simulink model "Mech_sys_nl_obs_deformation"  (R2025b)
settings: Solver=ode15s  StartTime=0.0  StopTime=10.0  RelTol=1e-3
values from neighbouring files (symbols this model uses):
  p_0 = 0    [Init_Simulink_param.m]
  phat_0 = 1e-3    (= 0.001)    [Init_Simulink_param.m]
  q_0 = 0    [Init_Simulink_param.m]
  qhat_0 = 2e-4    (= 0.0002)    [Init_Simulink_param.m]
undefined symbols (not defined in the file or in its folder): params
settings Model: Creator=filippougolini  LastModifiedBy=filippougolini

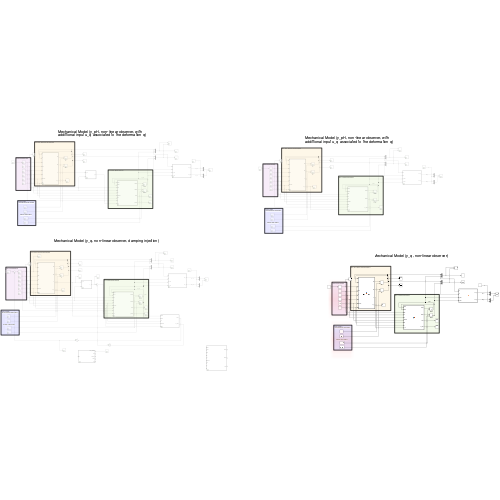
[thumbnail: Simulink's stored preview of the top-level diagram]
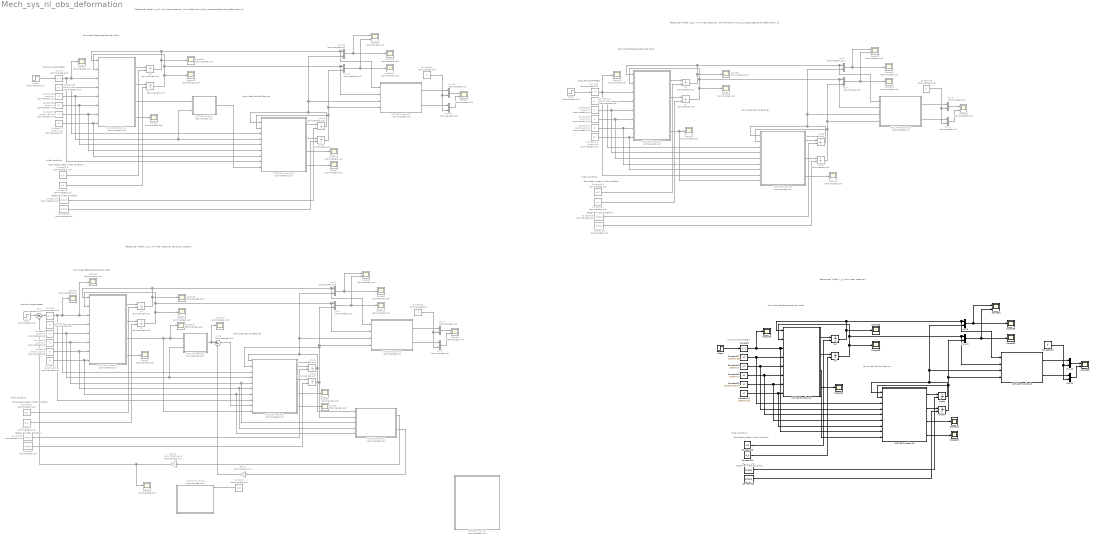
== system Mech_sys_nl_obs_deformation ==
  note: Non-linear Electromechanical plant
  note: Observer initial condition
  note: Non-Linear Spirito Oberver
  note: NonLinear system initial condition
  note: Mechanical Model (y_pH, non-linear observer, with addittional input u_q associated to the deformation q)
  note: Input and parameters
  note: Initial condition
  note: Mechanical Model (y_q, non-linear observer, damping injection)
  note: Non-Linear Spirito Oberver
  note: NonLinear system initial condition
  note: Input and parameters
  note: Initial condition
  note: Non-linear Electromechanical plant
  note: Observer initial condition
  note: Mechanical Model (y_pH, non-linear observer, with addittional input u_q associated to the deformation q)
  note: Non-Linear Spirito Oberver
  note: NonLinear system initial condition
  note: Input and parameters
  note: Initial condition
  note: Non-linear Electromechanical plant
  note: Observer initial condition
  note: NonLinear system initial condition
  note: Non-Linear Spirito Oberver
  note: Observer initial condition
  note: Non-linear Electromechanical plant
  note: Initial condition
  note: Mechanical Model (y_q, non-linear observer)
  note: Input and parameters
  Constant : Constant  Commented=on  Value=100
  Constant1 : Constant  Commented=on  Value=params.q0
  Constant10 : Constant  Commented=on  Value=params.m
  Constant11 : Constant  Commented=on  Value=params.q0
  Constant12 : Constant  Commented=on  Value=params.epsllon
  Constant13 : Constant  Commented=on  Value=q_0
  Constant14 : Constant  Commented=on  Value=p_0
  Constant15 : Constant  Commented=on  Value=qhat_0
  Constant16 : Constant  Commented=on  Value=phat_0
  Constant17 : Constant  Commented=on  Value=params.eta
  Constant18 : Constant  Commented=on  Value=0
  Constant19 : Constant  Commented=on  Value=params.K
  Constant2 : Constant  Commented=on  Value=params.epsllon
  Constant20 : Constant  Commented=on  Value=params.m
  Constant21 : Constant  Value=params.q0
  Constant22 : Constant  Value=params.epsllon
  Constant23 : Constant  Value=q_0
  Constant24 : Constant  Value=p_0
  Constant25 : Constant  Value=qhat_0
  Constant26 : Constant  Value=phat_0
  Constant27 : Constant  Value=params.eta
  Constant28 : Constant  Value=0
  Constant29 : Constant  Value=params.K
  Constant3 : Constant  Commented=on  Value=q_0
  Constant30 : Constant  Value=params.m
  Constant4 : Constant  Commented=on  Value=p_0
  Constant5 : Constant  Commented=on  Value=qhat_0
  Constant6 : Constant  Commented=on  Value=phat_0
  Constant7 : Constant  Commented=on  Value=10
  Constant71 : Constant  Commented=on  Value=params.q0
  Constant74 : Constant  Commented=on  Value=params.epsllon
  Constant76 : Constant  Commented=on  Value=q_0
  Constant77 : Constant  Commented=on  Value=p_0
  Constant79 : Constant  Commented=on  Value=qhat_0
  Constant8 : Constant  Commented=on  Value=0
  Constant80 : Constant  Commented=on  Value=phat_0
  Constant85 : Constant  Commented=on  Value=params.eta
  Constant9 : Constant  Commented=on  Value=params.K
  Constant90 : Constant  Commented=on  Value=0
  Constant92 : Constant  Commented=on  Value=params.K
  Constant93 : Constant  Commented=on  Value=params.m
  Gain1 : Gain  Commented=on  Gain=0
  Gain2 : Gain  Commented=on  Gain=4.957213974e13
  MATLAB Function : MATLAB Function  Commented=on  TreatAsAtomicUnit=on
  MATLAB Function1 : MATLAB Function  Commented=on  TreatAsAtomicUnit=on
  MATLAB Function10 : MATLAB Function  Commented=on  TreatAsAtomicUnit=on
  MATLAB Function12 : MATLAB Function  TreatAsAtomicUnit=on
  MATLAB Function13 : MATLAB Function  TreatAsAtomicUnit=on
  MATLAB Function14 : MATLAB Function  Commented=on  TreatAsAtomicUnit=on
  MATLAB Function15 : MATLAB Function  TreatAsAtomicUnit=on
  MATLAB Function18 : MATLAB Function  Commented=on  TreatAsAtomicUnit=on
  MATLAB Function2 : MATLAB Function  Commented=on  TreatAsAtomicUnit=on
  MATLAB Function22 : MATLAB Function  Commented=on  TreatAsAtomicUnit=on
  MATLAB Function3 : MATLAB Function  Commented=on  TreatAsAtomicUnit=on
  MATLAB Function4 : MATLAB Function  Commented=on  TreatAsAtomicUnit=on
  MATLAB Function5 : MATLAB Function  Commented=on  TreatAsAtomicUnit=on
  MATLAB Function6 : MATLAB Function  Commented=on  TreatAsAtomicUnit=on
  MATLAB Function7 : MATLAB Function  Commented=on  TreatAsAtomicUnit=on
  MATLAB Function8 : MATLAB Function  Commented=on  TreatAsAtomicUnit=on
  MATLAB Function9 : MATLAB Function  Commented=on  TreatAsAtomicUnit=on
  Mux{1..8,39..40,44,46} (12 alike) : Mux  Commented=on  Inputs=2
  Mux{9..12} (4 alike) : Mux  Inputs=2
  Scope{1..7,9..10,12..19,21..22,24..25,27..28,43..44,52..53} (27 alike) : Scope  Commented=on
      Scope1 settings: ActiveDisplayYMinimum=-1  ActiveDisplayYMaximum=1
      Scope10 settings: ActiveDisplayYMinimum=-1  ActiveDisplayYMaximum=1  DataLoggingVariableName=ScopeData3
      Scope12 settings: ActiveDisplayYMinimum=-4.0944874698701246E-5  ActiveDisplayYMaximum=0.0003685038722883113  DataLoggingVariableName=ScopeData5
      Scope13 settings: ActiveDisplayYMinimum=999.83794210721385  ActiveDisplayYMaximum=1000.4797286758781  DataLoggingVariableName=ScopeData12
      Scope14 settings: ActiveDisplayYMinimum=-1  ActiveDisplayYMaximum=1  DataLoggingVariableName=ScopeData6
      Scope15 settings: ActiveDisplayYMinimum=2.4999952064993516E+7  ActiveDisplayYMaximum=2.5000040184962828E+7  DataLoggingVariableName=ScopeData14
      Scope16 settings: ActiveDisplayYMinimum=-3.6994045804858762E+6  ActiveDisplayYMaximum=3.9014912238323367E+6  DataLoggingVariableName=ScopeData15
      Scope17 settings: ActiveDisplayYMinimum=-4.9067926815122174E-14  ActiveDisplayYMaximum=5.0932073184877836E-14  DataLoggingVariableName=ScopeData16
      Scope18 settings: ActiveDisplayYMinimum=-1  ActiveDisplayYMaximum=1  DataLoggingVariableName=ScopeData17
      Scope19 settings: ActiveDisplayYMinimum=-1  ActiveDisplayYMaximum=1  DataLoggingVariableName=ScopeData18
      Scope2 settings: ActiveDisplayYMinimum=-4.486759019288802E-5  ActiveDisplayYMaximum=0.00036893672106914937
      Scope21 settings: ActiveDisplayYMinimum=-4.486759019288802E-5  ActiveDisplayYMaximum=0.00036893672106914937  DataLoggingVariableName=ScopeData20
      Scope22 settings: ActiveDisplayYMinimum=0.000327102944393571  ActiveDisplayYMaximum=0.00032809892974007158  DataLoggingVariableName=ScopeData21
      Scope24 settings: ActiveDisplayYMinimum=-4.4929456410290065E-5  ActiveDisplayYMaximum=0.00036894675529116814  DataLoggingVariableName=ScopeData23
      Scope25 settings: ActiveDisplayYMinimum=-1  ActiveDisplayYMaximum=1  DataLoggingVariableName=ScopeData24
      Scope27 settings: ActiveDisplayYMinimum=-4.0944874698701246E-5  ActiveDisplayYMaximum=0.0003685038722883113  DataLoggingVariableName=ScopeData26
      Scope28 settings: ActiveDisplayYMinimum=-1  ActiveDisplayYMaximum=1  DataLoggingVariableName=ScopeData27
      Scope3 settings: ActiveDisplayYMinimum=-1  ActiveDisplayYMaximum=1  DataLoggingVariableName=ScopeData2
      Scope4 settings: ActiveDisplayYMinimum=-1  ActiveDisplayYMaximum=1  DataLoggingVariableName=ScopeData7
      Scope43 settings: ActiveDisplayYMinimum=-4.4929456410290065E-5  ActiveDisplayYMaximum=0.00036894675529116814  DataLoggingVariableName=ScopeData43
      Scope44 settings: ActiveDisplayYMinimum=-1  ActiveDisplayYMaximum=1  DataLoggingVariableName=ScopeData44
      Scope5 settings: ActiveDisplayYMinimum=-3.6994045804858764E-11  ActiveDisplayYMaximum=3.9014912238323363E-11  DataLoggingVariableName=ScopeData8
      Scope52 settings: ActiveDisplayYMinimum=-4.0944874698701246E-5  ActiveDisplayYMaximum=0.0003685038722883113  DataLoggingVariableName=ScopeData52
      Scope53 settings: ActiveDisplayYMinimum=-1  ActiveDisplayYMaximum=1  DataLoggingVariableName=ScopeData53
      Scope6 settings: ActiveDisplayYMinimum=-4.486759019288802E-5  ActiveDisplayYMaximum=0.00036893672106914937  DataLoggingVariableName=ScopeData9
      Scope7 settings: ActiveDisplayYMinimum=-1  ActiveDisplayYMaximum=1  DataLoggingVariableName=ScopeData10
      Scope9 settings: ActiveDisplayYMinimum=-4.4929456410290065E-5  ActiveDisplayYMaximum=0.00036894675529116814  DataLoggingVariableName=ScopeData13
  Scope{8,11,23,26,37,47} (6 alike) : Scope  Commented=on  NumInputPorts=2
      Scope11 settings: ActiveDisplayYMinimum=-1.6721224120479319E-8  ActiveDisplayYMaximum=1.6255351844579E-8  DataLoggingVariableName=ScopeData4
      Scope23 settings: ActiveDisplayYMinimum=-0.0031018408255779882  ActiveDisplayYMaximum=0.0026704507247831775  DataLoggingVariableName=ScopeData22
      Scope26 settings: ActiveDisplayYMinimum=-0.0014405764588177341  ActiveDisplayYMaximum=0.0029651881293596056  DataLoggingVariableName=ScopeData25
      Scope37 settings: ActiveDisplayYMinimum=-0.0033069856482364551  ActiveDisplayYMaximum=0.0026922054561645506  DataLoggingVariableName=ScopeData37
      Scope47 settings: ActiveDisplayYMinimum=-0.0014633833172245443  ActiveDisplayYMaximum=0.0031704498550208992  DataLoggingVariableName=ScopeData47
      Scope8 settings: ActiveDisplayYMinimum=-0.0048034948171394934  ActiveDisplayYMaximum=0.0043294231290401794  DataLoggingVariableName=ScopeData11
  Scope{20,29..31,33..34,36,38} (8 alike) : Scope
      Scope20 settings: ActiveDisplayYMinimum=-1  ActiveDisplayYMaximum=1  DataLoggingVariableName=ScopeData19
      Scope29 settings: ActiveDisplayYMinimum=-2.6358030258124043E-11  ActiveDisplayYMaximum=1.925982917121927E-11  DataLoggingVariableName=ScopeData28
      Scope30 settings: ActiveDisplayYMinimum=0.0003271907516113819  ActiveDisplayYMaximum=0.00032820530698062  DataLoggingVariableName=ScopeData29
      Scope31 settings: ActiveDisplayYMinimum=-4.0944150570938618E-5  ActiveDisplayYMaximum=0.00036849735513844764  DataLoggingVariableName=ScopeData30
      Scope33 settings: ActiveDisplayYMinimum=-4.4929456410290065E-5  ActiveDisplayYMaximum=0.00036894675529116814  DataLoggingVariableName=ScopeData32
      Scope34 settings: ActiveDisplayYMinimum=-1  ActiveDisplayYMaximum=1  DataLoggingVariableName=ScopeData33
      Scope36 settings: ActiveDisplayYMinimum=0.00032749819334930381  ActiveDisplayYMaximum=0.0003276391478829251  DataLoggingVariableName=ScopeData35
      Scope38 settings: ActiveDisplayYMinimum=-1  ActiveDisplayYMaximum=1  DataLoggingVariableName=ScopeData36
  Scope32 : Scope  NumInputPorts=2
      settings: ActiveDisplayYMinimum=-0.0033241234591442474  ActiveDisplayYMaximum=0.0028464455936065003  DataLoggingVariableName=ScopeData31
  Scope35 : Scope  NumInputPorts=2
      settings: ActiveDisplayYMinimum=-0.0014633833192336466  ActiveDisplayYMaximum=0.0031704498731028193  DataLoggingVariableName=ScopeData34
  Square : Math  Commented=on  Operator=square
  Square1 : Math  Commented=on  Operator=square
  Square2 : Math  Commented=on  Operator=square
  Square3 : Math  Operator=square
  Step1 : Step  Commented=on  After=5e3  SampleTime=0
  Step2 : Step  Commented=on  After=5e3  SampleTime=0
  Step3 : Step  Commented=on  After=5e3  SampleTime=0
  Step4 : Step  After=5e3  SampleTime=0
  Sum : Sum  Commented=on  Inputs=|+-
  Sum1 : Sum  Commented=on  Inputs=|+-
  p1 : Integrator  Commented=on  InitialConditionSource=external
  p2 : Integrator  Commented=on  InitialConditionSource=external
  p3 : Integrator  Commented=on  InitialConditionSource=external
  p4 : Integrator  InitialConditionSource=external
  phat1 : Integrator  Commented=on  InitialConditionSource=external  InitialCondition=5e-4
  phat2 : Integrator  Commented=on  InitialConditionSource=external  InitialCondition=5e-4
  phat3 : Integrator  Commented=on  InitialConditionSource=external  InitialCondition=5e-4
  phat4 : Integrator  InitialConditionSource=external  InitialCondition=5e-4
  q1 : Integrator  Commented=on  InitialConditionSource=external
  q2 : Integrator  Commented=on  InitialConditionSource=external
  q3 : Integrator  Commented=on  InitialConditionSource=external
  q4 : Integrator  InitialConditionSource=external
  qhat1 : Integrator  Commented=on  InitialConditionSource=external  InitialCondition=20e-5
  qhat2 : Integrator  Commented=on  InitialConditionSource=external  InitialCondition=20e-5
  qhat3 : Integrator  Commented=on  InitialConditionSource=external  InitialCondition=20e-5
  qhat4 : Integrator  InitialConditionSource=external  InitialCondition=20e-5
  wires:
  Step3/1 -> Square/1
  MATLAB Function18/3(yhat) -> Scope13/1
  MATLAB Function14/3(y) -> MATLAB Function/1(y_ph)
  Constant80/1 -> phat3/2
  Mux39/1 -> Scope37/1, Scope43/1
  Mux46/1 -> Scope47/1
  Mux40/1 -> Scope37/2, Scope44/1
  phat3/1 -> Mux40/2, MATLAB Function22/4(p_hat), MATLAB Function18/2(phat)  "p_hat"
  Constant93/1 -> MATLAB Function18/5(m), MATLAB Function14/6(m)
  MATLAB Function22/1(err_q) -> Mux46/1  "err_q"
  Constant79/1 -> qhat3/2
  Constant71/1 -> MATLAB Function18/7(q0), MATLAB Function14/8(q0)
  Constant92/1 -> MATLAB Function/2(K), MATLAB Function18/4(K), MATLAB Function14/5(K)
  Constant77/1 -> p3/2
  qhat3/1 -> Mux39/2, MATLAB Function22/3(q_hat), MATLAB Function18/1(qhat)  "q_hat"
  MATLAB Function18/2(dphat) -> phat3/1
  Constant85/1 -> MATLAB Function18/3(eta), MATLAB Function14/4(eta)
  Mux44/1 -> Scope47/2
  MATLAB Function14/1(dq) -> q3/1
  p3/1 -> Scope53/1, Mux40/1, MATLAB Function22/2(p), MATLAB Function14/2(p)  "p"
  MATLAB Function22/2(err_p) -> Mux44/1  "err_p"
  q3/1 -> Scope52/1, Mux39/1, MATLAB Function22/1(q), MATLAB Function14/1(q)  "q"
  MATLAB Function18/1(dqhat) -> qhat3/1
  Constant90/1 -> Mux44/2, Mux46/2  "0"
  Constant76/1 -> q3/2
  Constant74/1 -> MATLAB Function18/6(epsllon), MATLAB Function14/7(epsllon)
  MATLAB Function14/2(dp) -> p3/1
  Square/1 -> MATLAB Function18/8(u), MATLAB Function14/3(u), Scope1/1
  MATLAB Function/1(u_q) -> MATLAB Function18/9(u_q)
  MATLAB Function18/4(y_qhat) -> Scope2/1
  MATLAB Function14/4(y_q) -> Scope3/1
  Mux1/1 -> Scope8/1, Scope9/1
  Constant2/1 -> MATLAB Function3/6(epsllon), MATLAB Function5/4(epsllon), MATLAB Function2/7(epsllon)
  MATLAB Function2/4(y_q) -> Scope7/1
  Constant1/1 -> MATLAB Function3/7(q0), MATLAB Function5/5(q0), MATLAB Function2/8(q0)
  Constant7/1 -> MATLAB Function3/3(eta), MATLAB Function2/4(eta)
  MATLAB Function2/3(y) -> MATLAB Function3/10(y), Scope18/1, MATLAB Function1/1(y_ph)
  Mux2/1 -> Scope8/2, Scope10/1
  Constant10/1 -> MATLAB Function5/3(m), MATLAB Function3/5(m), MATLAB Function2/6(m)
  MATLAB Function3/4(y_qhat) -> Scope6/1
  Constant5/1 -> qhat1/2
  Constant3/1 -> q1/2
  p1/1 -> Scope14/1, Mux2/1, MATLAB Function4/2(p), MATLAB Function2/2(p)  "p"
  Constant6/1 -> phat1/2
  phat1/1 -> Mux2/2, MATLAB Function4/4(p_hat), MATLAB Function3/2(phat), MATLAB Function5/2(phat)  "p_hat"
  MATLAB Function4/1(err_q) -> Mux4/1  "err_q"
  Constant9/1 -> MATLAB Function1/2(K), MATLAB Function3/4(K), MATLAB Function2/5(K)
  qhat1/1 -> Mux1/2, MATLAB Function4/3(q_hat), MATLAB Function3/1(qhat), MATLAB Function5/1(qhat)  "q_hat"
  MATLAB Function2/1(dq) -> q1/1
  MATLAB Function4/2(err_p) -> Mux3/1  "err_p"
  MATLAB Function3/3(yhat) -> Scope5/1
  MATLAB Function3/1(dqhat) -> qhat1/1
  Constant8/1 -> Mux3/2, Mux4/2  "0"
  MATLAB Function2/2(dp) -> p1/1
  Mux4/1 -> Scope11/1
  Constant4/1 -> p1/2
  MATLAB Function3/2(dphat) -> phat1/1
  Mux3/1 -> Scope11/2
  q1/1 -> Scope12/1, Mux1/1, MATLAB Function4/1(q), MATLAB Function2/1(q)  "q"
  Square1/1 -> MATLAB Function3/8(u), MATLAB Function2/3(u), Scope15/1, Scope4/1
  Gain2/1 -> Sum/2, Scope16/1
  MATLAB Function5/1(yhat) -> Gain2/1
  MATLAB Function5/2(y_qhat) -> Gain1/1
  Gain1/1 -> Sum1/2
  MATLAB Function1/1(u_q) -> Scope17/1, Sum1/1
  Sum1/1 -> MATLAB Function3/9(u_q)
  Sum/1 -> Square1/1
  Step1/1 -> Sum/1
  Constant/1 -> MATLAB Function6/1(eta_original)
  Mux5/1 -> Scope23/1, Scope24/1
  Step2/1 -> Square2/1
  Constant12/1 -> MATLAB Function9/6(epsllon), MATLAB Function8/7(epsllon)
  MATLAB Function8/4(y_q) -> MATLAB Function9/9(y_q), Scope22/1
  Constant11/1 -> MATLAB Function9/7(q0), MATLAB Function8/8(q0)
  Constant17/1 -> MATLAB Function9/3(eta), MATLAB Function8/4(eta)
  Square2/1 -> MATLAB Function8/3(u), Scope19/1, MATLAB Function9/8(u)
  Mux6/1 -> Scope23/2, Scope25/1
  Constant20/1 -> MATLAB Function9/5(m), MATLAB Function8/6(m)
  MATLAB Function9/3(y_qhat) -> Scope21/1
  Constant15/1 -> qhat2/2
  Constant13/1 -> q2/2
  p2/1 -> Scope28/1, Mux6/1, MATLAB Function10/2(p), MATLAB Function8/2(p)  "p"
  Constant16/1 -> phat2/2
  phat2/1 -> Mux6/2, MATLAB Function10/4(p_hat), MATLAB Function9/2(phat)  "p_hat"
  MATLAB Function10/1(err_q) -> Mux8/1  "err_q"
  Constant19/1 -> MATLAB Function9/4(K), MATLAB Function8/5(K)
  qhat2/1 -> Mux5/2, MATLAB Function10/3(q_hat), MATLAB Function9/1(qhat)  "q_hat"
  MATLAB Function8/1(dq) -> q2/1
  MATLAB Function10/2(err_p) -> Mux7/1  "err_p"
  MATLAB Function9/1(dqhat) -> qhat2/1
  Constant18/1 -> Mux7/2, Mux8/2  "0"
  MATLAB Function8/2(dp) -> p2/1
  Mux8/1 -> Scope26/1
  Constant14/1 -> p2/2
  MATLAB Function9/2(dphat) -> phat2/1
  Mux7/1 -> Scope26/2
  q2/1 -> Scope27/1, Mux5/1, MATLAB Function10/1(q), MATLAB Function8/1(q)  "q"
  Constant28/1 -> Mux11/2, Mux12/2  "0"
  MATLAB Function13/1(dqhat) -> qhat4/1
  Mux12/1 -> Scope35/1
  Constant26/1 -> phat4/2
  Constant24/1 -> p4/2
  MATLAB Function13/2(dphat) -> phat4/1
  Square3/1 -> MATLAB Function13/8(u), MATLAB Function12/3(u), Scope20/1
  Constant30/1 -> MATLAB Function13/5(m), MATLAB Function12/6(m)
  Constant25/1 -> qhat4/2
  qhat4/1 -> Mux9/2, MATLAB Function15/3(q_hat), MATLAB Function13/1(qhat)  "q_hat"
  Mux9/1 -> Scope32/1, Scope33/1
  p4/1 -> Scope38/1, Mux10/1, MATLAB Function15/2(p), MATLAB Function12/2(p)  "p"
  MATLAB Function13/4(y_qhat) -> Scope30/1
  phat4/1 -> Mux10/2, MATLAB Function15/4(p_hat), MATLAB Function13/2(phat)  "p_hat"
  Constant27/1 -> MATLAB Function13/3(eta), MATLAB Function12/4(eta)
  Step4/1 -> Square3/1
  MATLAB Function15/2(err_p) -> Mux11/1  "err_p"
  Constant23/1 -> q4/2
  MATLAB Function13/3(yhat) -> Scope29/1
  MATLAB Function15/1(err_q) -> Mux12/1  "err_q"
  Mux10/1 -> Scope32/2, Scope34/1
  Constant21/1 -> MATLAB Function13/7(q0), MATLAB Function12/8(q0)
  Mux11/1 -> Scope35/2
  MATLAB Function12/2(dp) -> p4/1
  q4/1 -> Scope36/1, Mux9/1, MATLAB Function15/1(q), MATLAB Function12/1(q)  "q"
  Constant22/1 -> MATLAB Function13/6(epsllon), MATLAB Function12/7(epsllon)
  MATLAB Function12/1(dq) -> q4/1
  MATLAB Function12/4(y_q) -> Scope31/1
  Constant29/1 -> MATLAB Function13/4(K), MATLAB Function12/5(K)
  MATLAB Function12/3(y) -> MATLAB Function13/9(y_q)

== matlab function Mech_sys_nl_obs_deformation/MATLAB Function10 ==
  data: q input; err_q output; p input; q_hat input; p_hat input; err_p output
function [err_q, err_p] = error(q, p, q_hat, p_hat)

    err_q = q - q_hat;
    err_p = p - p_hat;
end

== matlab function Mech_sys_nl_obs_deformation/MATLAB Function7 ==
  data: qhat input; phat input; eta input; K input; m input; epsllon input; q0 input; u input; dqhat output; y input; dphat output; yhat output
function [dqhat, dphat, yhat] = observer_pH_mech_yph(qhat, phat, ...
    eta, K, m, epsllon, q0, u, y)

    % Port-Hamiltonian structure matrices
    J = [  0  1;
          -1  0 ];

    R = diag([0, eta]);
    g = [0; 2*epsllon*(qhat + q0)^3];

    % dH/dqhat
    dHhdqh = K*qhat;
    % dH/dphat
    dHhdph = phat / m;
    % dH/dQhat

    gradHh = [dHhdqh; dHhdph];
    % L = [0, 20*2*epsllon*(qhat + q0)^3];
    L = [0, 20];

    % -------- Observer gain L --------
    Lcol = L.';       % ensure it's 3x1

    yhat = 2*(phat / m)*epsllon*(qhat + q0)^3;

    % -------- Observer dynamics --------
    % Note: J and R are constant
    xhatdot = (J - R) * gradHh + g*u + Lcol * (y - yhat);

    dqhat = xhatdot(1);
    dphat = xhatdot(2);
end

== matlab function Mech_sys_nl_obs_deformation/MATLAB Function8 ==
  data: q input; p input; u input; dq output; eta input; K input; m input; epsllon input; q0 input; dp output; y output; y_q output
function [dq, dp, y, y_q] = plant_pH_mech(q, p, u, eta, K, m, epsllon, q0)
% Electro-mechanical pH plant

    % Parameters: m, K, eta, eps, re, q0 in workspace

    J = [  0  1 ;
          -1  0 ];

    R = diag([0, eta]);
    g = [0; 2*epsllon*(q + q0)^3];

    dHdq = K * q;
    dHdp = p / m;

    gradH = [dHdq; dHdp];

    xdot = (J - R) * gradH + g*u;

    y = 2*(p / m)*epsllon*(q + q0)^3;

    psi_T = [1/K, 0];
    y_q = psi_T * gradH;

    
    dq = xdot(1);
    dp = xdot(2);
end

== matlab function Mech_sys_nl_obs_deformation/MATLAB Function9 ==
  data: qhat input; phat input; eta input; K input; m input; epsllon input; q0 input; u input; dqhat output; dphat output; y_q input; y_qhat output
function [dqhat, dphat, y_qhat] = observer_pH_mech_yph(qhat, phat, ...
    eta, K, m, epsllon, q0, u, y_q)

    % Port-Hamiltonian structure matrices
    J = [  0  1;
          -1  0 ];

    R = diag([0, eta]);
    g = [0; 2*epsllon*(qhat + q0)^3];

    % dH/dqhat
    dHhdqh = K*qhat;
    % dH/dphat
    dHhdph = phat / m;
    % dH/dQhat

    gradHh = [dHhdqh; dHhdph];
    % L = [0, 20*2*epsllon*(qhat + q0)^3];
    L = [0, 20];

    % -------- Observer gain L --------
    Lcol = L.';       % ensure it's 3x1

    %yhat = 2*(phat / m)*epsllon*(qhat + q0)^3;
    psi = [1/K, 0];
    y_qhat = psi * gradHh;
    % -------- Observer dynamics --------
    % Note: J and R are constant
    xhatdot = (J - R) * gradHh + g*u  - Lcol*(y_q - y_qhat);
    % xhatdot = (J - R) * gradHh + g*u;

    dqhat = xhatdot(1);
    dphat = xhatdot(2);
end

== matlab function Mech_sys_nl_obs_deformation/MATLAB Function12 ==
  data: q input; p input; u input; dq output; eta input; K input; m input; epsllon input; q0 input; dp output; y output; y_q output
function [dq, dp, y, y_q] = plant_pH_mech(q, p, u, eta, K, m, epsllon, q0)
% Electro-mechanical pH plant

    % Parameters: m, K, eta, eps, re, q0 in workspace

    J = [  0  1 ;
          -1  0 ];

    R = diag([0, eta]);
    g = [0; 2*epsllon*(q + q0)^3];

    dHdq = K * q;
    dHdp = p / m;

    gradH = [dHdq; dHdp];

    xdot = (J - R) * gradH + g*u;

    y = 2*(p / m)*epsllon*(q + q0)^3;

    psi_T = [1/K, 0];
    y_q = psi_T * gradH;

    
    dq = xdot(1);
    dp = xdot(2);
end

== matlab function Mech_sys_nl_obs_deformation/MATLAB Function13 ==
  data: qhat input; phat input; eta input; K input; m input; epsllon input; q0 input; u input; dqhat output; dphat output; yhat output; y_qhat output; y_q input
function [dqhat, dphat, yhat, y_qhat] = observer_pH_mech_yph(qhat, phat, ...
    eta, K, m, epsllon, q0, u, y_q)

    % Port-Hamiltonian structure matrices
    J = [  0  1;
          -1  0 ];

    R = diag([0, eta]);
    g = [0; 2*epsllon*(qhat + q0)^3];

    % dH/dqhat
    dHhdqh = K*qhat;
    % dH/dphat
    dHhdph = phat / m;
    % dH/dQhat

    gradHh = [dHhdqh; dHhdph];
    % L = [0, 20*2*epsllon*(qhat + q0)^3];
    L = [0, 20];

    % -------- Observer gain L --------
    Lcol = L.';       % ensure it's 3x1

    yhat = 2*(phat / m)*epsllon*(qhat + q0)^3;
    psi = [1/K, 0];
    % -------- Observer dynamics --------
    % Note: J and R are constant
    xhatdot = (J - R) * gradHh + g*u  - Lcol*(y_q - yhat);
    y_qhat = psi * gradHh;

    dqhat = xhatdot(1);
    dphat = xhatdot(2);
end

== matlab function Mech_sys_nl_obs_deformation/MATLAB Function14 ==
  data: q input; p input; u input; dq output; eta input; K input; m input; epsllon input; q0 input; dp output; y output; y_q output
function [dq, dp, y, y_q] = plant_pH_mech(q, p, u, eta, K, m, epsllon, q0)
% Electro-mechanical pH plant

    % Parameters: m, K, eta, eps, re, q0 in workspace

    J = [  0  1 ;
          -1  0 ];

    R = diag([0, eta]);
    g = [0; 2*epsllon*(q + q0)^3];

    dHdq = K * q;
    dHdp = p / m;

    gradH = [dHdq; dHdp];

    xdot = (J - R) * gradH + g*u;

    y = 2*(p / m)*epsllon*(q + q0)^3;

    psi_T = [1/K, 0];
    y_q = psi_T * gradH;

    
    dq = xdot(1);
    dp = xdot(2);
end

== matlab function Mech_sys_nl_obs_deformation/MATLAB Function15 ==
  data: q input; err_q output; p input; q_hat input; p_hat input; err_p output
function [err_q, err_p] = error(q, p, q_hat, p_hat)

    err_q = q - q_hat;
    err_p = p - p_hat;
end

== matlab function Mech_sys_nl_obs_deformation/MATLAB Function18 ==
  data: qhat input; phat input; eta input; K input; m input; epsllon input; q0 input; u input; dqhat output; dphat output; yhat output; u_q input; y_qhat output
function [dqhat, dphat, yhat, y_qhat] = observer_pH_mech_yph(qhat, phat, ...
    eta, K, m, epsllon, q0, u, u_q)

    % Port-Hamiltonian structure matrices
    J = [  0  1;
          -1  0 ];

    R = diag([0, eta]);
    g = [0; 2*epsllon*(qhat + q0)^3];

    % dH/dqhat
    dHhdqh = K*qhat;
    % dH/dphat
    dHhdph = phat / m;
    % dH/dQhat

    gradHh = [dHhdqh; dHhdph];
    % L = [0, 20*2*epsllon*(qhat + q0)^3];
    L = [0, 20];

    % -------- Observer gain L --------
    Lcol = L.';       % ensure it's 3x1

    yhat = 2*(phat / m)*epsllon*(qhat + q0)^3;
    psi = [1/K, 0];
    % -------- Observer dynamics --------
    % Note: J and R are constant
    xhatdot = (J - R) * gradHh + g*u  - Lcol*yhat + psi*u_q;
    y_qhat = psi * gradHh;

    dqhat = xhatdot(1);
    dphat = xhatdot(2);
end

== matlab function Mech_sys_nl_obs_deformation/MATLAB Function1 ==
  data: y_ph input; K input; u_q output
function u_q = fcn(y_ph, K)

psi_T = [1/K, 0];
right_pse_psi = [K, 0];
L = [0, 20];

u_q = right_pse_psi * L' * y_ph;

end

== matlab function Mech_sys_nl_obs_deformation/MATLAB Function22 ==
  data: q input; err_q output; p input; q_hat input; p_hat input; err_p output
function [err_q, err_p] = error(q, p, q_hat, p_hat)

    err_q = q - q_hat;
    err_p = p - p_hat;
end

== matlab function Mech_sys_nl_obs_deformation/MATLAB Function ==
  data: y_ph input; K input; u_q output
function u_q = fcn(y_ph, K)

psi_T = [1/K, 0];
right_pse_psi = [K, 0];
L = [0, 20];

u_q = right_pse_psi * L' * y_ph;

end

== matlab function Mech_sys_nl_obs_deformation/MATLAB Function2 ==
  data: q input; p input; u input; dq output; eta input; K input; m input; epsllon input; q0 input; dp output; y output; y_q output
function [dq, dp, y, y_q] = plant_pH_mech(q, p, u, eta, K, m, epsllon, q0)
% Electro-mechanical pH plant

    % Parameters: m, K, eta, eps, re, q0 in workspace

    J = [  0  1 ;
          -1  0 ];

    R = diag([0, eta]);
    g = [0; 2*epsllon*(q + q0)^3];

    dHdq = K * q;
    dHdp = p / m;

    gradH = [dHdq; dHdp];

    xdot = (J - R) * gradH + g*u;

    y = 2*(p / m)*epsllon*(q + q0)^3;

    psi_T = [1/K, 0];
    y_q = psi_T * gradH;

    
    dq = xdot(1);
    dp = xdot(2);
end

== matlab function Mech_sys_nl_obs_deformation/MATLAB Function3 ==
  data: qhat input; phat input; eta input; K input; m input; epsllon input; q0 input; u input; dqhat output; dphat output; yhat output; u_q input; y_qhat output; y input
function [dqhat, dphat, yhat, y_qhat] = observer_pH_mech_yph(qhat, phat, ...
    eta, K, m, epsllon, q0, u, u_q, y)

    % Port-Hamiltonian structure matrices
    J = [  0  1;
          -1  0 ];

    R = diag([0, eta]);
    g = [0; 2*epsllon*(qhat + q0)^3];

    % dH/dqhat
    dHhdqh = K*qhat;
    % dH/dphat
    dHhdph = phat / m;
    % dH/dQhat

    gradHh = [dHhdqh; dHhdph];
    % L = [0, 20*2*epsllon*(qhat + q0)^3];
    L = [0, 20];

    % -------- Observer gain L --------
    Lcol = L.';       % ensure it's 3x1

    yhat = 2*(phat / m)*epsllon*(qhat + q0)^3;
    psi = [1/K, 0];
    % -------- Observer dynamics --------
    % Note: J and R are constant
    % xhatdot = (J - R) * gradHh + g*u  - Lcol*yhat + psi*u_q;
    xhatdot = (J - R) * gradHh + g*u  - Lcol*(y - yhat);

    y_qhat = psi * gradHh;

    dqhat = xhatdot(1);
    dphat = xhatdot(2);
end

== matlab function Mech_sys_nl_obs_deformation/MATLAB Function4 ==
  data: q input; err_q output; p input; q_hat input; p_hat input; err_p output
function [err_q, err_p] = error(q, p, q_hat, p_hat)

    err_q = q - q_hat;
    err_p = p - p_hat;
end

== matlab function Mech_sys_nl_obs_deformation/MATLAB Function5 ==
  data: qhat input; yhat output; phat input; m input; epsllon input; q0 input; y_qhat output
function [yhat, y_qhat] = fcn(qhat, phat, m, epsllon, q0)

    yhat = 2*(phat / m)*epsllon*(qhat + q0)^3;
    y_qhat = qhat;
end

== matlab function Mech_sys_nl_obs_deformation/MATLAB Function6 ==
  data: eta_original input; Kd output; eta input; epsllon input; qhat input; q0 input
function Kd = fcn(eta_original, eta, epsllon, qhat, q0)

    Kd = (eta_original - eta)/(8*epsllon^2*(qhat + q0)^6);

end
